simulink model "DC_motor_controller_tram_sim"  (R2023a)
settings: Solver=ode23t  StartTime=0.0  StopTime=800  RelTol=1e-3
values from neighbouring files (symbols this model uses):
  En = P_mecc/ia_n    (= 540)    [DC_motor_controller_tram.m]
  g = 9.81    [DC_motor_controller_tram.m]
  Ga = 1/Ra/(1+tau_a*s)    [DC_motor_controller_tram.m]
  Ge = 1/Re/(1+tau_e*s)    [DC_motor_controller_tram.m]
  Gm = 1/(J*s+beta)    [DC_motor_controller_tram.m]
  ie_n = 1    [DC_motor_controller_tram.m]
  K = En/w_n/ie_n    (= 1.71974522293)    [DC_motor_controller_tram.m]
  kb_ca = ki_ca/kp_ca    (= 100)    [DC_motor_controller_tram.m]
  kb_ce = ki_ce/kp_ce    (= 1)    [DC_motor_controller_tram.m]
  kb_v = ki_v/kp_v    (= 100)    [DC_motor_controller_tram.m]
  kb_w = ki_w/kp_w    (= 0.0133337883959)    [DC_motor_controller_tram.m]
  ki_ca = 42.06*2    (= 84.12)    [DC_motor_controller_tram.m]
  ki_ce = 120000    [DC_motor_controller_tram.m]
  ki_v = 10    [DC_motor_controller_tram.m]
  ki_w = 97.67    [DC_motor_controller_tram.m]
  kp_ca = 0.4206*2    (= 0.8412)    [DC_motor_controller_tram.m]
  kp_ce = 120000    [DC_motor_controller_tram.m]
  kp_v = 0.1    [DC_motor_controller_tram.m]
  kp_w = 7325    [DC_motor_controller_tram.m]
  PF = 1/(1+5.3*s)    [DC_motor_controller_tram.m]
  r = v_n_mps/w_n    (= 0.0530785562633)    [DC_motor_controller_tram.m]
  Ra = Va_n*(Va_n-En)/(Pel)    (= 0.0841153846154)    [DC_motor_controller_tram.m]
  V_supply = 600    [DC_motor_controller_tram.m]
  Ve_n = 120    [DC_motor_controller_tram.m]
libraries: slpidlib x4
settings Model: Creator=Andrea  LastModifiedBy=Andrea
settings OptimizationCC: ReuseModelBlockBuffer=off

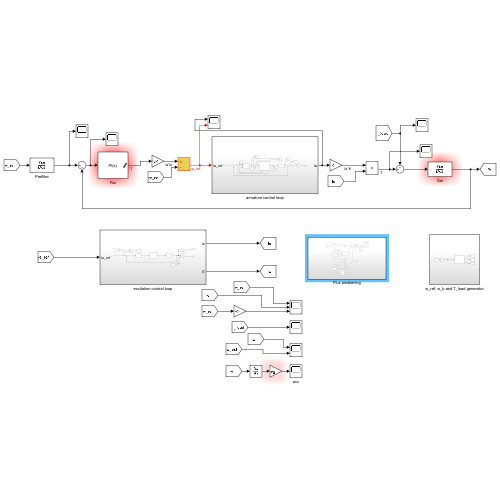
[thumbnail: Simulink's stored preview of the top-level diagram]
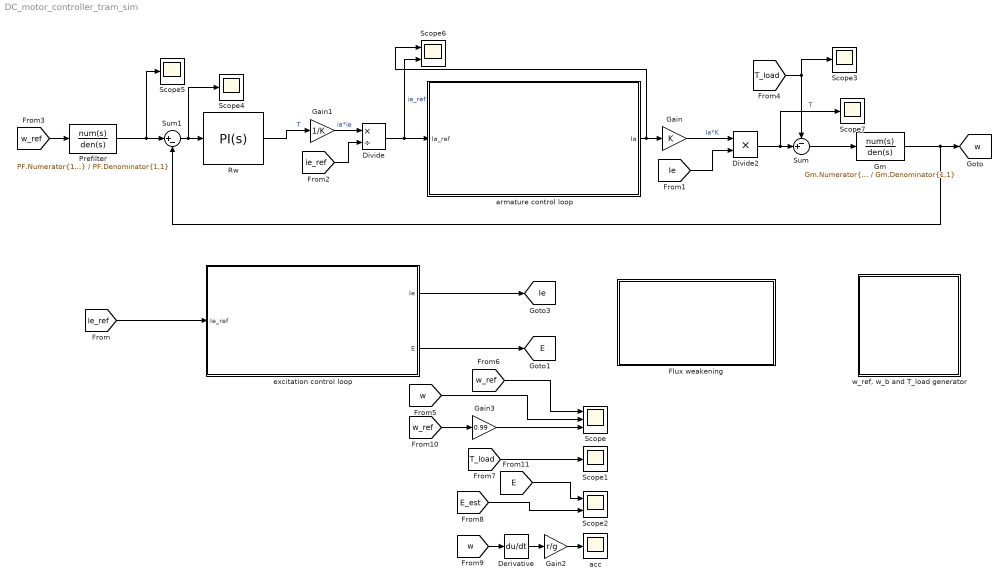
== system DC_motor_controller_tram_sim ==
  Derivative : Derivative
  Divide : Product  Inputs=*/  RndMeth=Zero  SaturateOnIntegerOverflow=on
  Divide2 : Product  Inputs=**  RndMeth=Zero  SaturateOnIntegerOverflow=on
  Flux weakening : Subsystem
  Gain : Gain  Gain=K
  Gain1 : Gain  Gain=1/K
  Gain2 : Gain  Gain=r/g
  Gain3 : Gain  Gain=0.99
  Gm : TransferFcn  Numerator=Gm.Numerator{1,1}  Denominator=Gm.Denominator{1,1}
  Prefilter : TransferFcn  Numerator=PF.Numerator{1,1}  Denominator=PF.Denominator{1,1}
  Rw : slpidlib/PID Controller  Controller=PI  Form=Parallel  TimeDomain=Continuous-time  UseExternalTs=off  SampleTime=-1  IntegratorMethod=Forward Euler  FilterMethod=Forward Euler  ControllerParametersSource=internal  P=kp_w  I=ki_w  UseKiTs=off  D=0  N=100  UseFilter=on  TunerSelectOption=Frequency Response Based  InitialConditionSource=internal  InitialConditionForIntegrator=0  InitialConditionForFilter=0  DifferentiatorICPrevScaledInput=0  ExternalReset=none  TrackingMode=off  Kt=1  LimitOutput=on  SatLimitsSource=internal  UpperSaturationLimit=10000  LowerSaturationLimit=-10000  LinearizeAsGain=on  AntiWindupMode=back-calculation  Kb=kb_w  LimitIntegrator=off  UpperIntegratorSaturationLimit=inf  LowerIntegratorSaturationLimit=-inf  POutMin=[]  POutMax=[]  IOutMin=[]  IOutMax=[]  DOutMin=[]  DOutMax=[]  NOutMin=[]  NOutMax=[]  SumOutMin=[]  SumOutMax=[]  SaturationOutMin=[]  SaturationOutMax=[]  PParamMin=[]  PParamMax=[]  IParamMin=[]  IParamMax=[]  DParamMin=[]  DParamMax=[]  NParamMin=[]  NParamMax=[]  KbParamMin=[]  KbParamMax=[]  KtParamMin=[]  KtParamMax=[]  KbOutMin=[]  KbOutMax=[]  KtOutMin=[]  KtOutMax=[]  IntegratorOutMin=[]  IntegratorOutMax=[]  FilterOutMin=[]  FilterOutMax=[]  SumI1OutMin=[]  SumI1OutMax=[]  SumI2OutMin=[]  SumI2OutMax=[]  SumI3OutMin=[]  SumI3OutMax=[]  SumI4OutMin=[]  SumI4OutMax=[]  SumDOutMin=[]  SumDOutMax=[]  DifferentiatorOutMin=[]  DifferentiatorOutMax=[]  FilterDiffOutCoefMin=[]  FilterDiffOutCoefMax=[]  ReciprocalOutMin=[]  ReciprocalOutMax=[]  SumDenOutMin=[]  SumDenOutMax=[]  SumNumOutMin=[]  SumNumOutMax=[]  DivideOutMin=[]  DivideOutMax=[]  UdiffTsProdOutMin=[]  UdiffTsProdOutMax=[]  NTsProdOutMin=[]  NTsProdOutMax=[]  UintegralTsProdOutMin=[]  UintegralTsProdOutMax=[]  UngainTsProdOutMin=[]  UngainTsProdOutMax=[]  ClampingZeroOutDataTypeStr=Inherit: Inherit via back propagation  ClampingZeroOutMin=[]  ClampingZeroOutMax=[]  FilterDenConstantOutDataTypeStr=Inherit: Inherit via back propagation  FilterDenConstantOutMin=[]  FilterDenConstantOutMax=[]  PCopyOutDataTypeStr=Inherit: Inherit via back propagation  PCopyOutMin=[]  PCopyOutMax=[]  NCopyOutDataTypeStr=Inherit: Inherit via back propagation  NCopyOutMin=[]  NCopyOutMax=[]  IntegratorContinuousStateAttributes=''  IntegratorStateMustResolveToSignalObject=off  IntegratorRTWStateStorageClass=Auto  FilterContinuousStateAttributes=''  FilterStateMustResolveToSignalObject=off  FilterRTWStateStorageClass=Auto  ParallelPVariant=InternalParameters  IdealPVariant=Disabled  IVariant=InternalParameters  DVariant=Disabled  IntegratorVariant=Continuous  SatVariant=Enabled  AWVariant=BackCalculation  PCopyVariant=Disabled  TRVariant=Disabled  FdbkBlocksVariant=Forward  IdealPFdbkVariant=Disabled  SatFdbkVariant=Disabled  DerivativeFilterVariant=Disabled  NVariant=Disabled  NCopyVariant=Disabled_SignalSpec  FilterICVariant=Disabled  IntegratorICVariant=InternalICs  ExternalResetVariant=Disabled  TRSumVariant=Passthrough  SumFdbkVariant=Disabled  SumVariant=Sum_PI  TsampFilterVariant=InternalTs  TsampNgainVariant=Passthrough  TsampIntegralVariant=Disabled_SignalSpec  ExternalSaturationOutDataTypeStr=Inherit: Same as second input
  Scope : Scope  NumInputPorts=3
  Scope{1,3..5,7} (5 alike) : Scope
  Scope2 : Scope  NumInputPorts=2
  Scope6 : Scope  NumInputPorts=2
  Sum : Sum  Inputs=-+|
  Sum1 : Sum  Inputs=|+-
  acc : Scope
  armature control loop : Subsystem
  excitation control loop : Subsystem
  "w_ref, w_b and T_load generator" : Subsystem
  tag scope: E=global, Ie=global, w=global
  wires:
  Sum/1 -> Gm/1
  armature control loop/1(Ia) -> Scope6/1, Gain/1
  Gain/1 -> Divide2/1  "Ia*K"
  [Ie] -> Divide2/2
  excitation control loop/2(E) -> [E]
  excitation control loop/1(Ie) -> [Ie]
  [ie_ref] -> excitation control loop/1(Ie_ref)
  Gain1/1 -> Divide/1  "ia*ie"
  Divide/1 -> Scope6/2, armature control loop/1(Ia_ref)  "ia_ref"
  [ie_ref] -> Divide/2
  Sum1/1 -> Scope4/1, Rw/1
  Gm/1 -> Sum1/2, [w]
  [w_ref] -> Prefilter/1
  [T_load] -> Sum/1, Scope3/1
  [w] -> Scope/2
  [w_ref] -> Scope/1
  [T_load] -> Scope1/1
  Rw/1 -> Gain1/1  "T"
  [E_est] -> Scope2/2
  [w] -> Derivative/1
  Derivative/1 -> Gain2/1
  Gain2/1 -> acc/1
  Divide2/1 -> Scope7/1, Sum/2  "T"
  Prefilter/1 -> Scope5/1, Sum1/1
  [w_ref] -> Gain3/1
  Gain3/1 -> Scope/3
  [E] -> Scope2/1

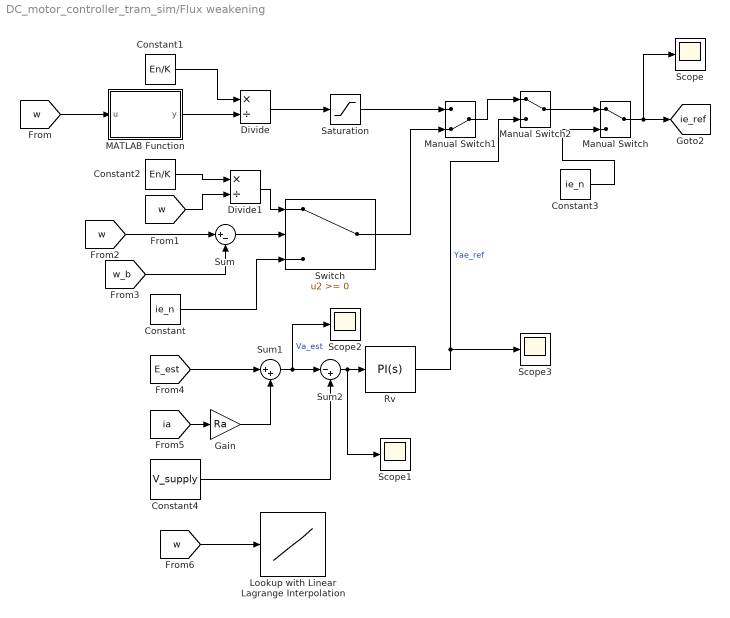
== system DC_motor_controller_tram_sim/Flux weakening ==
  Constant : Constant  Value=ie_n
  Constant1 : Constant  Value=En/K
  Constant2 : Constant  Value=En/K
  Constant3 : Constant  Value=ie_n
  Constant4 : Constant  Value=V_supply
  Divide : Product  Inputs=*/  RndMeth=Zero  SaturateOnIntegerOverflow=on
  Divide1 : Product  Inputs=*/  RndMeth=Zero  SaturateOnIntegerOverflow=on
  Gain : Gain  Gain=Ra
  Lookup with Linear Lagrange Interpolation : Lookup_n-D  NumberOfTableDimensions=1  BreakpointsForDimension1=[-5:5]  Table=tanh([-5:5])  InterpMethod=Linear Lagrange  InternalRulePriority=Speed  RndMeth=Simplest
  MATLAB Function : MATLAB Function  TreatAsAtomicUnit=on
  Manual Switch : ManualSwitch
  Manual Switch1 : ManualSwitch  CurrentSetting=0
  Manual Switch2 : ManualSwitch
  Rv : slpidlib/PID Controller  Controller=PI  Form=Parallel  TimeDomain=Continuous-time  UseExternalTs=off  SampleTime=-1  IntegratorMethod=Forward Euler  FilterMethod=Forward Euler  ControllerParametersSource=internal  P=kp_v  I=ki_v  UseKiTs=off  D=0  N=100  UseFilter=on  TunerSelectOption=Transfer Function Based (PID Tuner App)  InitialConditionSource=internal  InitialConditionForIntegrator=0  InitialConditionForFilter=0  DifferentiatorICPrevScaledInput=0  ExternalReset=none  TrackingMode=off  Kt=1  LimitOutput=on  SatLimitsSource=internal  UpperSaturationLimit=ie_n  LowerSaturationLimit=-ie_n  LinearizeAsGain=on  AntiWindupMode=back-calculation  Kb=kb_v  LimitIntegrator=off  UpperIntegratorSaturationLimit=inf  LowerIntegratorSaturationLimit=-inf  POutMin=[]  POutMax=[]  IOutMin=[]  IOutMax=[]  DOutMin=[]  DOutMax=[]  NOutMin=[]  NOutMax=[]  SumOutMin=[]  SumOutMax=[]  SaturationOutMin=[]  SaturationOutMax=[]  PParamMin=[]  PParamMax=[]  IParamMin=[]  IParamMax=[]  DParamMin=[]  DParamMax=[]  NParamMin=[]  NParamMax=[]  KbParamMin=[]  KbParamMax=[]  KtParamMin=[]  KtParamMax=[]  KbOutMin=[]  KbOutMax=[]  KtOutMin=[]  KtOutMax=[]  IntegratorOutMin=[]  IntegratorOutMax=[]  FilterOutMin=[]  FilterOutMax=[]  SumI1OutMin=[]  SumI1OutMax=[]  SumI2OutMin=[]  SumI2OutMax=[]  SumI3OutMin=[]  SumI3OutMax=[]  SumI4OutMin=[]  SumI4OutMax=[]  SumDOutMin=[]  SumDOutMax=[]  DifferentiatorOutMin=[]  DifferentiatorOutMax=[]  FilterDiffOutCoefMin=[]  FilterDiffOutCoefMax=[]  ReciprocalOutMin=[]  ReciprocalOutMax=[]  SumDenOutMin=[]  SumDenOutMax=[]  SumNumOutMin=[]  SumNumOutMax=[]  DivideOutMin=[]  DivideOutMax=[]  UdiffTsProdOutMin=[]  UdiffTsProdOutMax=[]  NTsProdOutMin=[]  NTsProdOutMax=[]  UintegralTsProdOutMin=[]  UintegralTsProdOutMax=[]  UngainTsProdOutMin=[]  UngainTsProdOutMax=[]  ClampingZeroOutDataTypeStr=Inherit: Inherit via back propagation  ClampingZeroOutMin=[]  ClampingZeroOutMax=[]  FilterDenConstantOutDataTypeStr=Inherit: Inherit via back propagation  FilterDenConstantOutMin=[]  FilterDenConstantOutMax=[]  PCopyOutDataTypeStr=Inherit: Inherit via back propagation  PCopyOutMin=[]  PCopyOutMax=[]  NCopyOutDataTypeStr=Inherit: Inherit via back propagation  NCopyOutMin=[]  NCopyOutMax=[]  IntegratorContinuousStateAttributes=''  IntegratorStateMustResolveToSignalObject=off  IntegratorRTWStateStorageClass=Auto  FilterContinuousStateAttributes=''  FilterStateMustResolveToSignalObject=off  FilterRTWStateStorageClass=Auto  ParallelPVariant=InternalParameters  IdealPVariant=Disabled  IVariant=InternalParameters  DVariant=Disabled  IntegratorVariant=Continuous  SatVariant=Enabled  AWVariant=BackCalculation  PCopyVariant=Disabled  TRVariant=Disabled  FdbkBlocksVariant=Forward  IdealPFdbkVariant=Disabled  SatFdbkVariant=Disabled  DerivativeFilterVariant=Disabled  NVariant=Disabled  NCopyVariant=Disabled_SignalSpec  FilterICVariant=Disabled  IntegratorICVariant=InternalICs  ExternalResetVariant=Disabled  TRSumVariant=Passthrough  SumFdbkVariant=Disabled  SumVariant=Sum_PI  TsampFilterVariant=InternalTs  TsampNgainVariant=Passthrough  TsampIntegralVariant=Disabled_SignalSpec  ExternalSaturationOutDataTypeStr=Inherit: Same as second input
  Saturation : Saturate  UpperLimit=ie_n  LowerLimit=-ie_n
  Scope{,1..3} (4 alike) : Scope
  Sum : Sum  Inputs=|+-
  Sum1 : Sum  Inputs=|++
  Sum2 : Sum  Inputs=|-+
  Switch : Switch  SaturateOnIntegerOverflow=off  InputSameDT=off
  tag scope: ie_ref=global
  wires:
  Constant1/1 -> Divide/1
  Divide/1 -> Saturation/1
  Constant2/1 -> Divide1/1
  [w] -> Divide1/2
  Divide1/1 -> Switch/1
  Constant/1 -> Switch/3
  Sum/1 -> Switch/2
  [w] -> Sum/1
  [w_b] -> Sum/2
  Constant3/1 -> Manual Switch/2
  [E_est] -> Sum1/1
  [ia] -> Gain/1
  Gain/1 -> Sum1/2
  Sum1/1 -> Scope2/1, Sum2/1  "Va_est"
  Constant4/1 -> Sum2/2
  Sum2/1 -> Scope1/1, Rv/1
  Saturation/1 -> Manual Switch1/1
  Switch/1 -> Manual Switch1/2
  Manual Switch/1 -> Scope/1, [ie_ref]
  MATLAB Function/1(y) -> Divide/2
  [w] -> MATLAB Function/1(u)
  Rv/1 -> Scope3/1, Manual Switch2/2  "Yae_ref"
  Manual Switch2/1 -> Manual Switch/1
  Manual Switch1/1 -> Manual Switch2/1
  [w] -> Lookup with Linear Lagrange Interpolation/1

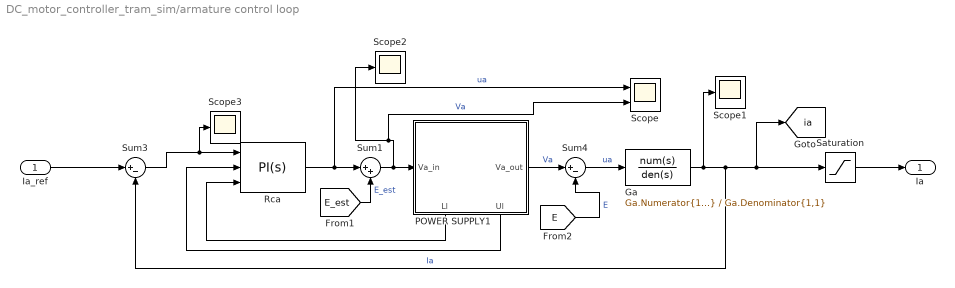
== system DC_motor_controller_tram_sim/armature control loop ==
  Ia_ref : Inport
  Ga : TransferFcn  Numerator=Ga.Numerator{1,1}  Denominator=Ga.Denominator{1,1}
  POWER SUPPLY1 : Subsystem
      settings: PortSchema="{\"entries\":[{\"content\":{\"sides\":[{\"content\":{\"connectorIds\":[\"In1\"]},\"type\":\"ConnectorPlacement.EquallySpacedRectSide\",\"uuid\":\"93eeac49-7421-40d0-9ee5-8ad57e829cd3\"},{\"content\":{\"connectorIds\":[\"Out1\"],\"side\":\"RIGHT\"},\"type\":\"ConnectorPlacement.EquallySpacedRectSide\",\"uuid\":\"5b0c3d71-2678-4b93-93e5-40fa5eeb5fbf\"},{\"content\":{\"connectorIds\":[],\"side\":\"TOP\"},\"type\":\"ConnectorPlacement.EquallySpacedRectSide\",\"uuid\":\"2461063a-90cb-4d9a-ae55-232c5bd72d76\"},{\"content\":{\"connectorIds\":[\"Out2\",\"Out3\"],\"side\":\"BOTTOM\"},\"type\":\"ConnectorPlacement.EquallySpacedRectSide\",\"uuid\":\"fa1dd5d5-6ed9-4f85-8e4e-36ee5927f3ce\"}]},\"type\":\"ConnectorPlacement.EquallySpacedConnector\",\"uuid\":\"b3d451a9-c46c-4a75-9bfc-93d300db0bd5\"}],\"packageUris\":[\"http://schema.mathworks.com/mf0/Connector/R2020b\"],\"version\":\"1.0\"}"
  Rca : slpidlib/PID Controller  Controller=PI  Form=Parallel  TimeDomain=Continuous-time  UseExternalTs=off  SampleTime=-1  IntegratorMethod=Forward Euler  FilterMethod=Forward Euler  ControllerParametersSource=internal  P=kp_ca  I=ki_ca  UseKiTs=off  D=0  N=100  UseFilter=on  TunerSelectOption=Transfer Function Based (PID Tuner App)  InitialConditionSource=internal  InitialConditionForIntegrator=0  InitialConditionForFilter=0  DifferentiatorICPrevScaledInput=0  ExternalReset=none  TrackingMode=off  Kt=1  LimitOutput=on  SatLimitsSource=external  UpperSaturationLimit=Ve_n  LowerSaturationLimit=-Ve_n  LinearizeAsGain=on  AntiWindupMode=back-calculation  Kb=kb_ca  LimitIntegrator=off  UpperIntegratorSaturationLimit=inf  LowerIntegratorSaturationLimit=-inf  POutMin=[]  POutMax=[]  IOutMin=[]  IOutMax=[]  DOutMin=[]  DOutMax=[]  NOutMin=[]  NOutMax=[]  SumOutMin=[]  SumOutMax=[]  SaturationOutMin=[]  SaturationOutMax=[]  PParamMin=[]  PParamMax=[]  IParamMin=[]  IParamMax=[]  DParamMin=[]  DParamMax=[]  NParamMin=[]  NParamMax=[]  KbParamMin=[]  KbParamMax=[]  KtParamMin=[]  KtParamMax=[]  KbOutMin=[]  KbOutMax=[]  KtOutMin=[]  KtOutMax=[]  IntegratorOutMin=[]  IntegratorOutMax=[]  FilterOutMin=[]  FilterOutMax=[]  SumI1OutMin=[]  SumI1OutMax=[]  SumI2OutMin=[]  SumI2OutMax=[]  SumI3OutMin=[]  SumI3OutMax=[]  SumI4OutMin=[]  SumI4OutMax=[]  SumDOutMin=[]  SumDOutMax=[]  DifferentiatorOutMin=[]  DifferentiatorOutMax=[]  FilterDiffOutCoefMin=[]  FilterDiffOutCoefMax=[]  ReciprocalOutMin=[]  ReciprocalOutMax=[]  SumDenOutMin=[]  SumDenOutMax=[]  SumNumOutMin=[]  SumNumOutMax=[]  DivideOutMin=[]  DivideOutMax=[]  UdiffTsProdOutMin=[]  UdiffTsProdOutMax=[]  NTsProdOutMin=[]  NTsProdOutMax=[]  UintegralTsProdOutMin=[]  UintegralTsProdOutMax=[]  UngainTsProdOutMin=[]  UngainTsProdOutMax=[]  ClampingZeroOutDataTypeStr=Inherit: Inherit via back propagation  ClampingZeroOutMin=[]  ClampingZeroOutMax=[]  FilterDenConstantOutDataTypeStr=Inherit: Inherit via back propagation  FilterDenConstantOutMin=[]  FilterDenConstantOutMax=[]  PCopyOutDataTypeStr=Inherit: Inherit via back propagation  PCopyOutMin=[]  PCopyOutMax=[]  NCopyOutDataTypeStr=Inherit: Inherit via back propagation  NCopyOutMin=[]  NCopyOutMax=[]  IntegratorContinuousStateAttributes=''  IntegratorStateMustResolveToSignalObject=off  IntegratorRTWStateStorageClass=Auto  FilterContinuousStateAttributes=''  FilterStateMustResolveToSignalObject=off  FilterRTWStateStorageClass=Auto  ParallelPVariant=InternalParameters  IdealPVariant=Disabled  IVariant=InternalParameters  DVariant=Disabled  IntegratorVariant=Continuous  SatVariant=External  AWVariant=BackCalculation  PCopyVariant=Disabled  TRVariant=Disabled  FdbkBlocksVariant=Forward  IdealPFdbkVariant=Disabled  SatFdbkVariant=Disabled  DerivativeFilterVariant=Disabled  NVariant=Disabled  NCopyVariant=Disabled_SignalSpec  FilterICVariant=Disabled  IntegratorICVariant=InternalICs  ExternalResetVariant=Disabled  TRSumVariant=Passthrough  SumFdbkVariant=Disabled  SumVariant=Sum_PI  TsampFilterVariant=InternalTs  TsampNgainVariant=Passthrough  TsampIntegralVariant=Disabled_SignalSpec  ExternalSaturationOutDataTypeStr=Inherit: Same as second input
  Saturation : Saturate  UpperLimit=1000  LowerLimit=-1000
  Scope : Scope  NumInputPorts=2
  Scope1 : Scope
  Scope2 : Scope
  Scope3 : Scope
  Sum1 : Sum  Inputs=|++
  Sum3 : Sum  Inputs=|+-
  Sum4 : Sum  Inputs=|+-
  Ia : Outport
  tag scope: ia=global
  wires:
  [E_est] -> Sum1/2  "E_est"
  Sum1/1 -> Scope/2, Scope2/1, POWER SUPPLY1/1(Va_in)  "Va"
  Rca/1 -> Scope/1, Sum1/1  "ua"
  Ga/1 -> [ia], Saturation/1, Sum3/2, Scope1/1  "Ia"
  POWER SUPPLY1/3(Ul) -> Rca/2
  Sum4/1 -> Ga/1  "ua"
  POWER SUPPLY1/2(Ll) -> Rca/3
  Sum3/1 -> Scope3/1, Rca/1
  POWER SUPPLY1/1(Va_out) -> Sum4/1  "Va"
  [E] -> Sum4/2  "E"
  Ia_ref/1 -> Sum3/1
  Saturation/1 -> Ia/1

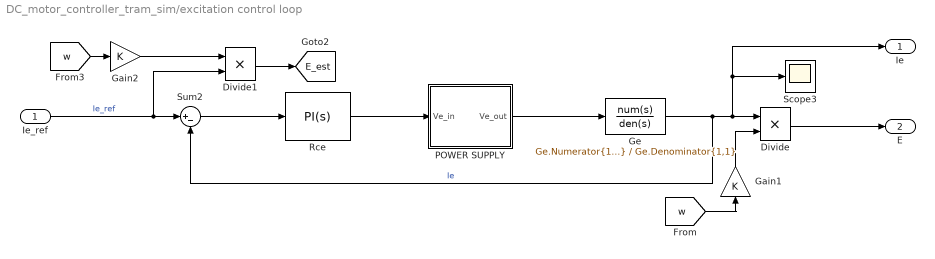
== system DC_motor_controller_tram_sim/excitation control loop ==
  Ie_ref : Inport
  Divide : Product  Inputs=**  RndMeth=Zero  SaturateOnIntegerOverflow=on
  Divide1 : Product  Inputs=**  RndMeth=Zero  SaturateOnIntegerOverflow=on
  Gain1 : Gain  Gain=K
  Gain2 : Gain  Gain=K
  Ge : TransferFcn  Numerator=Ge.Numerator{1,1}  Denominator=Ge.Denominator{1,1}
  POWER SUPPLY : Subsystem
  Rce : slpidlib/PID Controller  Controller=PI  Form=Parallel  TimeDomain=Continuous-time  UseExternalTs=off  SampleTime=-1  IntegratorMethod=Forward Euler  FilterMethod=Forward Euler  ControllerParametersSource=internal  P=kp_ce  I=ki_ce  UseKiTs=off  D=0  N=100  UseFilter=on  TunerSelectOption=Transfer Function Based (PID Tuner App)  InitialConditionSource=internal  InitialConditionForIntegrator=0  InitialConditionForFilter=0  DifferentiatorICPrevScaledInput=0  ExternalReset=none  TrackingMode=off  Kt=1  LimitOutput=on  SatLimitsSource=internal  UpperSaturationLimit=Ve_n  LowerSaturationLimit=-Ve_n  LinearizeAsGain=on  AntiWindupMode=back-calculation  Kb=kb_ce  LimitIntegrator=off  UpperIntegratorSaturationLimit=inf  LowerIntegratorSaturationLimit=-inf  POutMin=[]  POutMax=[]  IOutMin=[]  IOutMax=[]  DOutMin=[]  DOutMax=[]  NOutMin=[]  NOutMax=[]  SumOutMin=[]  SumOutMax=[]  SaturationOutMin=[]  SaturationOutMax=[]  PParamMin=[]  PParamMax=[]  IParamMin=[]  IParamMax=[]  DParamMin=[]  DParamMax=[]  NParamMin=[]  NParamMax=[]  KbParamMin=[]  KbParamMax=[]  KtParamMin=[]  KtParamMax=[]  KbOutMin=[]  KbOutMax=[]  KtOutMin=[]  KtOutMax=[]  IntegratorOutMin=[]  IntegratorOutMax=[]  FilterOutMin=[]  FilterOutMax=[]  SumI1OutMin=[]  SumI1OutMax=[]  SumI2OutMin=[]  SumI2OutMax=[]  SumI3OutMin=[]  SumI3OutMax=[]  SumI4OutMin=[]  SumI4OutMax=[]  SumDOutMin=[]  SumDOutMax=[]  DifferentiatorOutMin=[]  DifferentiatorOutMax=[]  FilterDiffOutCoefMin=[]  FilterDiffOutCoefMax=[]  ReciprocalOutMin=[]  ReciprocalOutMax=[]  SumDenOutMin=[]  SumDenOutMax=[]  SumNumOutMin=[]  SumNumOutMax=[]  DivideOutMin=[]  DivideOutMax=[]  UdiffTsProdOutMin=[]  UdiffTsProdOutMax=[]  NTsProdOutMin=[]  NTsProdOutMax=[]  UintegralTsProdOutMin=[]  UintegralTsProdOutMax=[]  UngainTsProdOutMin=[]  UngainTsProdOutMax=[]  ClampingZeroOutDataTypeStr=Inherit: Inherit via back propagation  ClampingZeroOutMin=[]  ClampingZeroOutMax=[]  FilterDenConstantOutDataTypeStr=Inherit: Inherit via back propagation  FilterDenConstantOutMin=[]  FilterDenConstantOutMax=[]  PCopyOutDataTypeStr=Inherit: Inherit via back propagation  PCopyOutMin=[]  PCopyOutMax=[]  NCopyOutDataTypeStr=Inherit: Inherit via back propagation  NCopyOutMin=[]  NCopyOutMax=[]  IntegratorContinuousStateAttributes=''  IntegratorStateMustResolveToSignalObject=off  IntegratorRTWStateStorageClass=Auto  FilterContinuousStateAttributes=''  FilterStateMustResolveToSignalObject=off  FilterRTWStateStorageClass=Auto  ParallelPVariant=InternalParameters  IdealPVariant=Disabled  IVariant=InternalParameters  DVariant=Disabled  IntegratorVariant=Continuous  SatVariant=Enabled  AWVariant=BackCalculation  PCopyVariant=Disabled  TRVariant=Disabled  FdbkBlocksVariant=Forward  IdealPFdbkVariant=Disabled  SatFdbkVariant=Disabled  DerivativeFilterVariant=Disabled  NVariant=Disabled  NCopyVariant=Disabled_SignalSpec  FilterICVariant=Disabled  IntegratorICVariant=InternalICs  ExternalResetVariant=Disabled  TRSumVariant=Passthrough  SumFdbkVariant=Disabled  SumVariant=Sum_PI  TsampFilterVariant=InternalTs  TsampNgainVariant=Passthrough  TsampIntegralVariant=Disabled_SignalSpec  ExternalSaturationOutDataTypeStr=Inherit: Same as second input
  Scope3 : Scope
  Sum2 : Sum  Inputs=|+-
  Ie : Outport
  E : Outport  Port=2
  tag scope: E_est=global
  wires:
  Ge/1 -> Ie/1, Scope3/1, Divide/1, Sum2/2  "Ie"
  Ie_ref/1 -> Divide1/2, Sum2/1  "Ie_ref"
  Sum2/1 -> Rce/1
  Divide/1 -> E/1
  Divide1/1 -> [E_est]
  [w] -> Gain1/1
  Gain2/1 -> Divide1/1
  [w] -> Gain2/1
  Gain1/1 -> Divide/2
  Rce/1 -> POWER SUPPLY/1(Ve_in)
  POWER SUPPLY/1(Ve_out) -> Ge/1

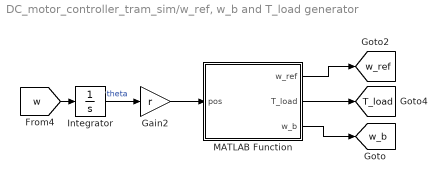
== system DC_motor_controller_tram_sim/w_ref, w_b and T_load generator ==
  Gain2 : Gain  Gain=r
  Integrator : Integrator
  MATLAB Function : MATLAB Function  TreatAsAtomicUnit=on
  tag scope: T_load=global, w_b=global, w_ref=global
  wires:
  Integrator/1 -> Gain2/1  "theta"
  [w] -> Integrator/1
  Gain2/1 -> MATLAB Function/1(pos)
  MATLAB Function/2(T_load) -> [T_load]
  MATLAB Function/1(w_ref) -> [w_ref]
  MATLAB Function/3(w_b) -> [w_b]

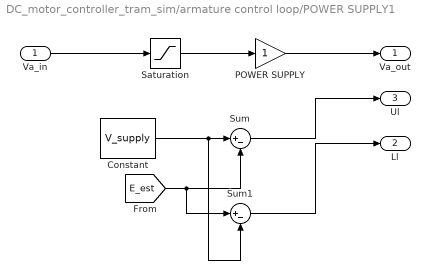
== system DC_motor_controller_tram_sim/armature control loop/POWER SUPPLY1 ==
  Va_in : Inport
  Constant : Constant  Value=V_supply
  POWER SUPPLY : Gain
  Saturation : Saturate  UpperLimit=V_supply  LowerLimit=-V_supply  LinearizeAsGain=off
  Sum : Sum  Inputs=|+-
  Sum1 : Sum  Inputs=|+-
  Va_out : Outport
  Ll : Outport  Port=2
  Ul : Outport  Port=3
  wires:
  POWER SUPPLY/1 -> Va_out/1
  Va_in/1 -> Saturation/1
  Saturation/1 -> POWER SUPPLY/1
  [E_est] -> Sum1/1, Sum/2
  Constant/1 -> Sum1/2, Sum/1
  Sum/1 -> Ul/1
  Sum1/1 -> Ll/1

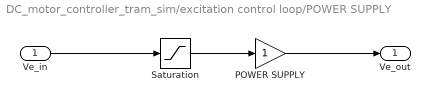
== system DC_motor_controller_tram_sim/excitation control loop/POWER SUPPLY ==
  Ve_in : Inport
  POWER SUPPLY : Gain
  Saturation : Saturate  UpperLimit=Ve_n  LowerLimit=-Ve_n
  Ve_out : Outport
  wires:
  Saturation/1 -> POWER SUPPLY/1
  Ve_in/1 -> Saturation/1
  POWER SUPPLY/1 -> Ve_out/1

== matlab function DC_motor_controller_tram_sim/w_ref, w_b and T_load generator/MATLAB Function ==
  data: pos input; w_ref output; T_load output; w_b output
function [w_ref,T_load, w_b]= fcn(pos)  
    %data
    v_n = 60;       % km/h
    w_n = 314;    %rad/s
    v_n_mps = v_n/3.6;
    r = v_n_mps/w_n;
    ts = 25;
    eta = 0.9;
    V_supply = 600;
    an = v_n_mps/ts;
    s_perc1 = 0;
    s_perc2 = 0;
    s_perc3 = 0.05;
    s_perc4 = 0;
    s_perc5 = 0;
    s_perc6 = -0.05;
    s_perc7 = 0;
    m_tram = 10e3;
    m_person = 80;
    n_people = 200;
    m_people = n_people*m_person;
    m_tot = m_tram+m_people;
    g = 9.81;
    Va_n = V_supply;
    ie_n = 1;
    F = m_tot*an;
    Ff = 1/3*F;
    Fn = F+Ff;
    Tn = Fn*r;
    Pn = Tn*w_n;
    Pel = Pn/eta;
    ia_n = Pel/Va_n;    
    En = Pn/ia_n;
    Ra = Va_n*(Va_n-En)/(Pel);
    beta = 1/3*Fn*v_n_mps/w_n^2;
    K = Tn/ie_n/ia_n;
    
    if pos <= 1000
        w_ref = 35/3.6/r;
        T_load = m_tot*g*r*sin(atan(s_perc1));
        w_b = (K*ie_n*V_supply/Ra-T_load)*1/(beta+K^2*ie_n^2/Ra); 
    elseif pos>1000 && pos<=3000
        w_ref = 60/3.6/r;
        T_load = m_tot*g*r*sin(atan(s_perc2));
        w_b = (K*ie_n*V_supply/Ra-T_load)*1/(beta+K^2*ie_n^2/Ra);
    elseif pos>3000 && pos<=4000
        w_ref = 60/3.6/r;
        T_load = m_tot*g*r*sin(atan(s_perc3));
        w_b = (K*ie_n*V_supply/Ra-T_load)*1/(beta+K^2*ie_n^2/Ra);
    elseif pos>4000 && pos<=6000
        w_ref = 75/3.6/r;
        T_load = m_tot*g*r*sin(atan(s_perc4));
        w_b = (K*ie_n*V_supply/Ra-T_load)*1/(beta+K^2*ie_n^2/Ra);
    elseif pos>6000 && pos<=8000
        w_ref = 60/3.6/r;
        T_load = m_tot*g*r*sin(atan(s_perc5));
        w_b = (K*ie_n*V_supply/Ra-T_load)*1/(beta+K^2*ie_n^2/Ra);
    elseif pos>8000 && pos<=9000
        w_ref = 60/3.6/r;
        T_load = m_tot*g*r*sin(atan(s_perc6));
        w_b = (K*ie_n*V_supply/Ra-T_load)*1/(beta+K^2*ie_n^2/Ra);
    elseif pos>9000 && pos<=10000
        w_ref = 35/3.6/r;
        T_load = m_tot*g*r*sin(atan(s_perc7));
        w_b = (K*ie_n*V_supply/Ra-T_load)*1/(beta+K^2*ie_n^2/Ra);
    else 
        w_ref = 0/3.6/r;
        T_load = m_tot*g*r*sin(atan(s_perc7));
        w_b = (K*ie_n*V_supply/Ra-T_load)*1/(beta+K^2*ie_n^2/Ra);
    end

== matlab function DC_motor_controller_tram_sim/Flux weakening/MATLAB Function ==
  data: u input; y output
function y = fcn(u)
    if u < 1
        y = 1;
    else
        y = u;
    end
